simulink model "continous_luenberger"  (R2020b)
settings: Solver=VariableStepAuto  StartTime=0.0  StopTime=10000  RelTol=1e-3
values from neighbouring files (symbols this model uses):
  A = [0 -theta2 0; 0 -1/theta3 1/theta3; 0 0 -1/theta3]    [script1.m]
  B = [0; 0; 1/theta3]    [script1.m]
  C = [1 0 0]    [script1.m]
  F_k = k*[1/theta2 -theta3 -theta3]    [script1.m]
undefined symbols (not defined in the file or in its folder): A_zoh, B_zoh, C_zoh, Gr, L, L_zoh, Ts
settings Model: SimulationMode=accelerator  Creator=Francesco  LastModifiedBy=Francesco

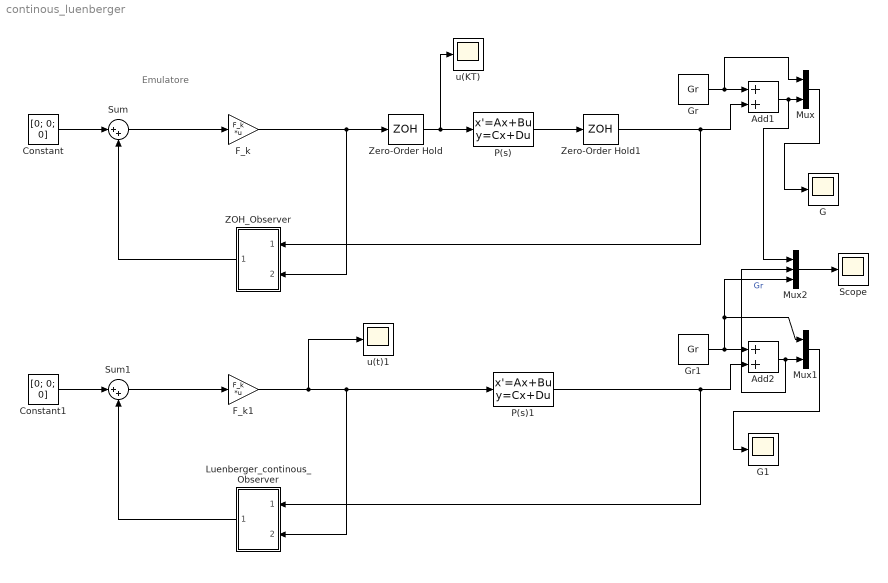
== system continous_luenberger ==
  note: Emulatore
  Add1 : Sum
  Add2 : Sum
  Constant : Constant  Value=[0; 0; 0]
  Constant1 : Constant  Value=[0; 0; 0]
  F_k : Gain  Gain=F_k  Multiplication=Matrix(K*u)
  F_k1 : Gain  Gain=F_k  Multiplication=Matrix(K*u)
  G : Scope
  G1 : Scope
  Gr : Constant  Value=Gr
  Gr1 : Constant  Value=Gr
  Luenberger_continous_Observer : Subsystem
  Mux : Mux  Inputs=2
  Mux1 : Mux  Inputs=2
  Mux2 : Mux  Inputs=3
  P(s) : StateSpace  A=A  B=B  C=C  D=0  InitialCondition=[130; 0; 0]
  P(s)1 : StateSpace  A=A  B=B  C=C  D=0  InitialCondition=[130; 0; 0]
  Scope : Scope
  Sum : Sum  Inputs=|++
  Sum1 : Sum  Inputs=|++
  ZOH_Observer : Subsystem
  Zero-Order Hold : ZeroOrderHold  SampleTime=Ts
  Zero-Order Hold1 : ZeroOrderHold  SampleTime=Ts
  u(KT) : Scope
  u(t)1 : Scope
  wires:
  P(s)/1 -> Zero-Order Hold1/1
  Mux/1 -> G/1
  Gr/1 -> Add1/1, Mux/1
  Add1/1 -> Mux2/1, Mux/2
  F_k/1 -> ZOH_Observer/2(In2), Zero-Order Hold/1
  Constant/1 -> Sum/1
  ZOH_Observer/1(Out1) -> Sum/2
  Zero-Order Hold/1 -> u(KT)/1, P(s)/1
  Zero-Order Hold1/1 -> ZOH_Observer/1(In1), Add1/2
  Sum/1 -> F_k/1
  Mux1/1 -> G1/1
  Gr1/1 -> Add2/1, Mux2/3, Mux1/1  "Gr"
  Add2/1 -> Mux2/2, Mux1/2
  P(s)1/1 -> Luenberger_continous_Observer/1(In1), Add2/2
  Luenberger_continous_Observer/1(Out1) -> Sum1/2
  Sum1/1 -> F_k1/1
  Constant1/1 -> Sum1/1
  F_k1/1 -> u(t)1/1, Luenberger_continous_Observer/2(In2), P(s)1/1
  Mux2/1 -> Scope/1

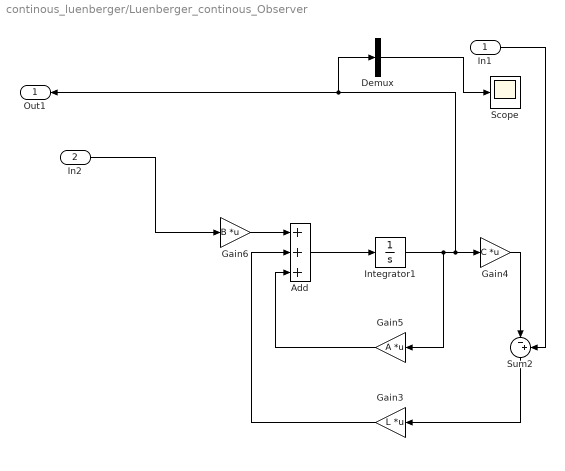
== system continous_luenberger/Luenberger_continous_Observer ==
  In1 : Inport
  In2 : Inport  Port=2
  Add : Sum  Inputs=+++
  Demux : Demux  Outputs=3
  Gain3 : Gain  Gain=L  Multiplication=Matrix(K*u)
  Gain4 : Gain  Gain=C  Multiplication=Matrix(K*u)
  Gain5 : Gain  Gain=A  Multiplication=Matrix(K*u)
  Gain6 : Gain  Gain=B  Multiplication=Matrix(K*u)
  Integrator1 : Integrator
  Scope : Scope
  Sum2 : Sum  Inputs=|-+
  Out1 : Outport
  wires:
  In1/1 -> Sum2/2
  Gain6/1 -> Add/1
  Sum2/1 -> Gain3/1
  Gain3/1 -> Add/2
  Gain4/1 -> Sum2/1
  Gain5/1 -> Add/3
  Add/1 -> Integrator1/1
  In2/1 -> Gain6/1
  Integrator1/1 -> Gain5/1, Demux/1, Out1/1, Gain4/1
  Demux/2 -> Scope/1

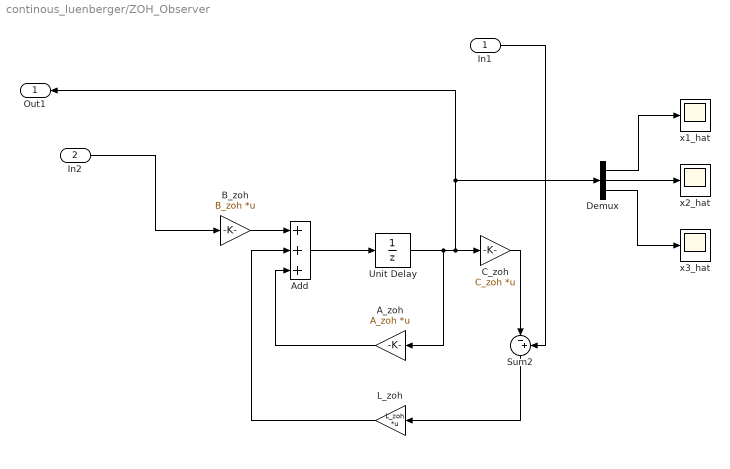
== system continous_luenberger/ZOH_Observer ==
  In1 : Inport
  In2 : Inport  Port=2
  A_zoh : Gain  Gain=A_zoh  Multiplication=Matrix(K*u)
  Add : Sum  Inputs=+++
  B_zoh : Gain  Gain=B_zoh  Multiplication=Matrix(K*u)
  C_zoh : Gain  Gain=C_zoh  Multiplication=Matrix(K*u)
  Demux : Demux  Outputs=3
  L_zoh : Gain  Gain=L_zoh  Multiplication=Matrix(K*u)
  Sum2 : Sum  Inputs=|-+
  Unit Delay : UnitDelay  SampleTime=-1  HasFrameUpgradeWarning=on
  x1_hat : Scope
  x2_hat : Scope
  x3_hat : Scope
  Out1 : Outport
  wires:
  In1/1 -> Sum2/2
  B_zoh/1 -> Add/1
  Sum2/1 -> L_zoh/1
  L_zoh/1 -> Add/2
  C_zoh/1 -> Sum2/1
  A_zoh/1 -> Add/3
  Add/1 -> Unit Delay/1
  In2/1 -> B_zoh/1
  Demux/1 -> x1_hat/1
  Unit Delay/1 -> A_zoh/1, Demux/1, Out1/1, C_zoh/1
  Demux/2 -> x2_hat/1
  Demux/3 -> x3_hat/1
